simulink model "FTTest01"  (R2013a)
settings: Solver=FixedStepDiscrete  StartTime=0.0  StopTime=10.0  FixedStep=0.001  RelTol=1e-3
settings Model: BufferReuse=off  Creator=bgbuss  LastModifiedBy=bgbuss
settings DataIOCC: LimitDataPoints=off
settings OptimizationCC: BlockReduction=off  OptimizeBlockIOStorage=off  BufferReuse=off  ExpressionFolding=off  LocalBlockOutputs=off
settings HardwareCC: ProdIntDivRoundTo=Zero  ProdEndianess=LittleEndian  ProdHWDeviceType=Generic->32-bit x86 compatible
settings RTWCC: SystemTargetFile=xpctarget.tlc  TemplateMakefile=xpc_default_tmf  Description=xPC Target  ProcessScript=xpctarget_make_rtw_hook  RTWCompilerOptimization=On
settings xpcTargetCC: TargetFcnLib=ansi_tfl_table_tmw.mat  CodeReplacementLibrary=XPC_BLAS  ParMdlRefBuildCompliant=on  ConcurrentExecutionCompliant=on  CombineSignalStateStructs=off  MATLABClassNameForMDSCustomization=xpcAperiodicCustomization  GRTInterface=on  GenerateAllocFcn=off  RL32LogBufSizeModifier=100000000  xPCTaskExecutionProfile=off  xPCRL32EventNumber=5000  xPCisModelTimeout=off  xPCModelTimeoutSecs=10  xPCLoadParamSetFile=off  xPCConcurrentTasks=off  xPCEnableSFAnimation=off

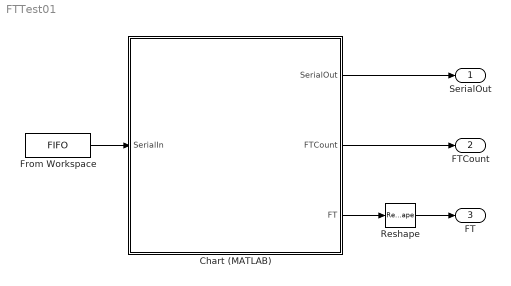
== system FTTest01 ==
  Chart (MATLAB) : Stateflow chart  TreatAsAtomicUnit=on
  From Workspace : FromWorkspace  VariableName=FIFO  SampleTime=0  Interpolate=off  OutputAfterFinalValue=Setting to zero
  Reshape : Reshape
  SerialOut : Outport
  FTCount : Outport  Port=2
  FT : Outport  Port=3
  wires:
  From Workspace/1 -> Chart (MATLAB)/1(SerialIn)
  Chart (MATLAB)/1(SerialOut) -> SerialOut/1
  Chart (MATLAB)/3(FT) -> Reshape/1
  Reshape/1 -> FT/1
  Chart (MATLAB)/2(FTCount) -> FTCount/1

== stateflow chart FTTest01/Chart (MATLAB) ==
  state InitializeStreaming
    en:
    SerialOut = [5; 10; 70; 85; 163; 157];
  state ParseStreaming
    en:
    SerialOut = [0; 0; 0; 0; 0; 0];
    SerialBufferEnd = 0;
    SerialBuffer = zeros(150,1,'uint8');
    du:
    parseStreamingData();
  (default) -> InitializeStreaming
  InitializeStreaming -> ParseStreaming
  data: SerialIn input size=101; SerialOut output size=6; SerialBuffer local uint8 size=150; SerialBufferEnd local size=1; FTCount output size=1; FT output size=[6 8]
  function parseStreamingData:
    | function parseStreamingData %#codegen
    |     % Insert the new data into the SerialBuffer
    |     numNewBytes = min(100, SerialIn(1));
    |     SerialBuffer(SerialBufferEnd + (1:numNewBytes)) = uint8(SerialIn(1 + (1:numNewBytes)));
    |     SerialBufferEnd = SerialBufferEnd + numNewBytes;
    |     FT = zeros(6,8);
    |     
    |     SerialBufferBegin = 1;
    |     FTCount = 0;
    |     k = 0;
    |     while k < SerialBufferEnd-12
    |         valid = CheckSample(SerialBuffer(k+(1:13)));
    |         if valid
    |             FTCount = FTCount + 1;
    |             FT(:,FTCount) = ComputeFT(SerialBuffer(k+(1:12)));
    |             k = k + 13;
    |             SerialBufferBegin = k + 1;
    |         else
    |             k = k + 1;
    |         end 
    |     end
    |     
    |     n = SerialBufferEnd - SerialBufferBegin + 1;
    |     SerialBuffer(1:n) = SerialBuffer(SerialBufferBegin:SerialBufferEnd);
    |     SerialBufferEnd = n;
    | end
    | 
    | function valid = CheckSample( sampleBytes )
    |     checkSum = uint16(0);
    |     for k = 1:12
    |         checkSum = checkSum + uint16(sampleBytes(k));
    |     end
    |     valid = bitand(checkSum, 127) == bitand(sampleBytes(13), 127);
    | end
    | 
    | function FT = ComputeFT(D)
    |     FT = double(D([1 3 5 7 9 11]))*256 + double(D([2 4 6 8 10 12]));
    |     %FT = double(D([1 3 5 7 9 11])) + double(D([2 4 6 8 10 12]))*256;
    | end
